simulink model "model_no_controller"  (R2016b)
settings: Solver=VariableStepAuto  StartTime=0.0  StopTime=10.0  RelTol=1e-3
values from neighbouring files (symbols this model uses):
  A = zeros(5,5)    [kalmanfilter.m]    (also in model_2017.m = [[0  0   0   0                0             0   1           ; model_rough.m; model_v2.m = [[0  0   0   0             0             0   1           0  ; model_v3.m = [[0  0   0   0                0             0   1           )
  B = zeros(5,6)    [kalmanfilter.m]    (also in model_2017.m = [[0      0      0      0     ];                        [0   ; model_rough.m; model_v2.m = [[0      0      0      0     ];                        [0   ; model_v3.m = [[0      0      0      0      0      0             ];       )
  C = eye(5)    [kalmanfilter.m]    (also in model_2017.m = [[0  0   0   0   0   0   1   0   0   0   0   0]; model_rough.m; model_v2.m = [[0  0   0   0   0   0   1   0   0   0   0   0]; model_v3.m = [[0  0   0   0   0   0   1   0   0   0   0   0])
settings Model: Creator=Simon's  LastModifiedBy=Simon's

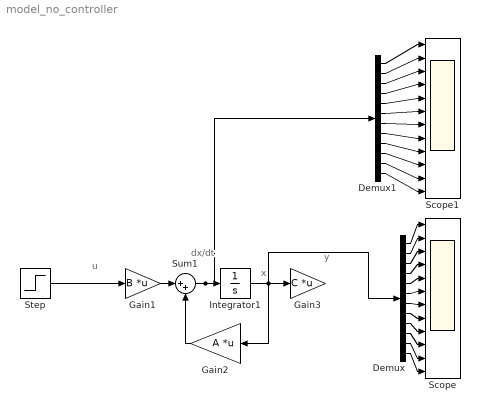
== system model_no_controller ==
  note: u
  note: y
  note: dx/dt
  note: x
  Demux : Demux  Outputs=12
  Demux1 : Demux  Outputs=12
  Gain1 : Gain  Gain=B  Multiplication=Matrix(K*u)
  Gain2 : Gain  Gain=A  Multiplication=Matrix(K*u)
  Gain3 : Gain  Gain=C  Multiplication=Matrix(K*u)
  Integrator1 : Integrator  InitialCondition=[0 0 0 0 0 0 0 0 0 0 0 0]'
  Scope : Scope  NumInputPorts=12
  Scope1 : Scope  NumInputPorts=12
  Step : Step  Before=[0 0 0 0]'  After=10*[0 0 1 1]'  SampleTime=0  VectorParams1D=off
  Sum1 : Sum  Inputs=|++
  wires:
  Gain1/1 -> Sum1/1
  Sum1/1 -> Demux1/1, Integrator1/1
  Gain2/1 -> Sum1/2
  Step/1 -> Gain1/1
  Integrator1/1 -> Demux/1, Gain2/1, Gain3/1
  Demux/1 -> Scope/1
  Demux/2 -> Scope/2
  Demux/3 -> Scope/3
  Demux/4 -> Scope/4
  Demux/5 -> Scope/5
  Demux/6 -> Scope/6
  Demux/7 -> Scope/7
  Demux/8 -> Scope/8
  Demux/9 -> Scope/9
  Demux/10 -> Scope/10
  Demux/11 -> Scope/11
  Demux/12 -> Scope/12
  Demux1/1 -> Scope1/1
  Demux1/2 -> Scope1/2
  Demux1/3 -> Scope1/3
  Demux1/4 -> Scope1/4
  Demux1/5 -> Scope1/5
  Demux1/6 -> Scope1/6
  Demux1/7 -> Scope1/7
  Demux1/8 -> Scope1/8
  Demux1/9 -> Scope1/9
  Demux1/10 -> Scope1/10
  Demux1/11 -> Scope1/11
  Demux1/12 -> Scope1/12
